simulink model "SimpleFlight"  (R2016b)
settings: Solver=ode4  StartTime=0.0  StopTime=inf  FixedStep=1/120  RelTol=1e-3  EnableMultiTasking=on
libraries: aerolibanimutils x2
settings Model: Creator=daspenc  LastModifiedBy=Zhanrui
settings DataIOCC: LimitDataPoints=on  SaveFormat=Array
settings OptimizationCC: LifeSpan=inf
settings DebuggingCC: UnderspecifiedInitializationDetection=Classic  MergeDetectMultiDrivingBlocksExec=none  SolverPrmCheckMsg=warning  AllowSymbolicDim=off  StateNameClashWarn=warning  SFUnexpectedBacktrackingDiag=warning  SFNoUnconditionalDefaultTransitionDiag=warning  SFExecutionAtInitializationDiag=none
settings HardwareCC: ProdBitPerPointer=32  ProdBitPerSizeT=32  ProdBitPerPtrDiffT=32  ProdLargestAtomicFloat=None  ProdIntDivRoundTo=Undefined  ProdEndianess=Unspecified  ProdWordSize=32  ProdHWDeviceType=32-bit Generic
settings ModelReferenceCC: PropagateSignalLabelsOutOfModel=off
settings GRTTargetCC: TargetLangStandard=C89/C90 (ANSI)  GeneratePreprocessorConditionals=Disable all
settings ConfigComp: CovMetricSettings=dw  CovHtmlReporting=on  CovSaveCumulativeToWorkspaceVar=on  CovSaveSingleToWorkspaceVar=on  CovExternalEMLEnable=off

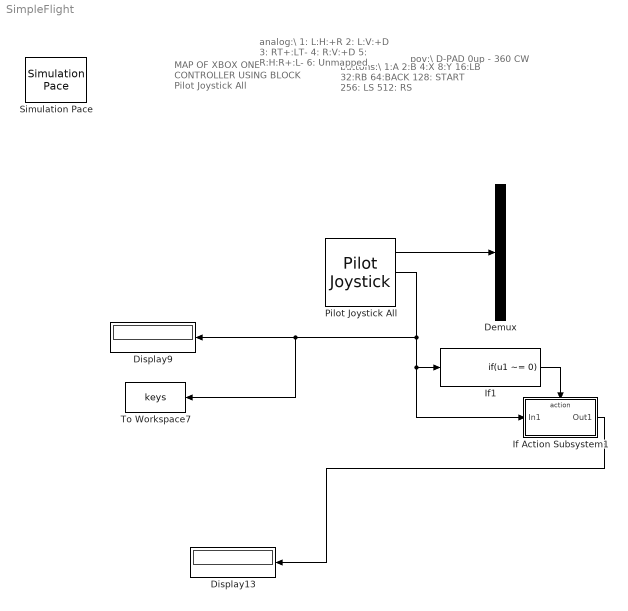
== system SimpleFlight ==
  note: MAP OF
      | XBOX ONE
      | CONTROLLER
      | USING BLOCK
      | Pilot Joystick All
  note: pov:\
      | D-PAD
      | 0up - 360 CW
  note: buttons:\
      | 1:A
      | 2:B
      | 4:X
      | 8:Y
      | 16:LB
      | 32:RB
      | 64:BACK
      | 128: START
      | 256: LS
      | 512: RS
  note: analog:\
      | 1: L:H:+R
      | 2: L:V:+D
      | 3: RT+:LT-
      | 4: R:V:+D
      | 5: R:H:R+:L-
      | 6: Unmapped
  Demux : Demux  Outputs=6
  Display13 : Display
  Display9 : Display
  If Action Subsystem1 : Subsystem  TreatAsAtomicUnit=on
  If1 : If  IfExpression=u1 ~= 0  ShowElse=off
  Pilot Joystick All : aerolibanimutils/Pilot Joystick  JoystickID=Joystick1  OutputConfiguration=AllOutputs  SampleTime=1/120
  Simulation Pace : aerolibanimutils/Simulation Pace  SimulationPace=1  SleepMode=MATLAB Thread  OutputPaceError=off  SampleTime=-1
      settings: AttributesFormatString=%<SimulationPace> sec/sec
  To Workspace7 : ToWorkspace  VariableName=keys  SaveFormat=Timeseries  SampleTime=-1
  wires:
  Pilot Joystick All/1 -> Demux/1
  If1/1 -> If Action Subsystem1/Action
  If Action Subsystem1/1(Out1) -> Display13/1
  Pilot Joystick All/2 -> Display9/1, To Workspace7/1, If1/1, If Action Subsystem1/1(In1)

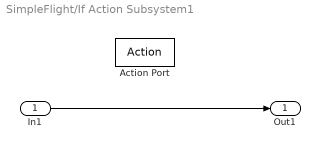
== system SimpleFlight/If Action Subsystem1 ==
  In1 : Inport
  Action Port : ActionPort  ActionType=then
  Out1 : Outport
  wires:
  In1/1 -> Out1/1
